simulink model "fpid_optimize_model"  (Simulink 7.5)
settings: Solver=ode23tb  StartTime=0.0  StopTime=100  FixedStep=0.5  RelTol=1e-3
libraries: cstblocks x2
settings Model: Creator=predoktor  LastModifiedBy=Alex
settings DataIOCC: LimitDataPoints=off  SignalLogging=off  DSMLogging=off  TimeSaveName=fpid_optimize_t  OutputSaveName=fpid_optimize_y

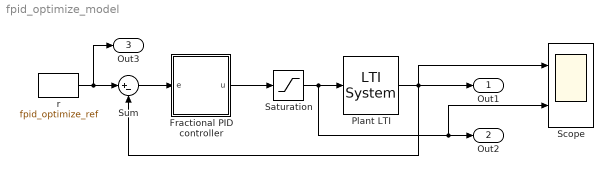
== system fpid_optimize_model ==
  Fractional PID controller : Subsystem
  Plant LTI : cstblocks/LTI System  SystemSampleTime=-1  sys=fpid_optimize_lti  IC=[]
  Saturation : Saturate  UpperLimit=Inf  LowerLimit=-Inf
  Scope : Scope  NumInputPorts=2
      settings: YMin=-5~-5  YMax=5~5
  Sum : Sum  Inputs=|+-
  r : FromWorkspace  VariableName=fpid_optimize_ref  SampleTime=0.5  Interpolate=off  OutputAfterFinalValue=Cyclic repetition
  Out1 : Outport
  Out2 : Outport  Port=2
  Out3 : Outport  Port=3
  wires:
  Sum/1 -> Fractional PID controller/1(e)
  Saturation/1 -> Out2/1, Scope/2, Plant LTI/1
  r/1 -> Out3/1, Sum/1
  Fractional PID controller/1(u) -> Saturation/1
  Plant LTI/1 -> Out1/1, Sum/2, Scope/1

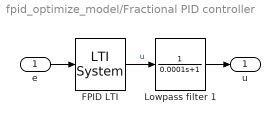
== system fpid_optimize_model/Fractional PID controller ==
  e : Inport
  FPID LTI : cstblocks/LTI System  SystemSampleTime=-1  sys=fpid_optimize_fpid  IC=[]
  Lowpass filter 1 : TransferFcn  Numerator=1  Denominator=[0.0001 1]
  u : Outport
  wires:
  FPID LTI/1 -> Lowpass filter 1/1  "u"
  e/1 -> FPID LTI/1
  Lowpass filter 1/1 -> u/1
